simulink model "mainprevius"  (R2024b)
settings: Solver=VariableStepAuto  StartTime=0.0  StopTime=20  RelTol=1e-3
undefined symbols (not defined in the file or in its folder): ZigBee
libraries: truetime x11, fuzblock x2
settings Model: PacingRate=2  Creator=giovanni02  LastModifiedBy=Utente
settings ConfigComp: CovBoundaryAbsTol=1.0e-5

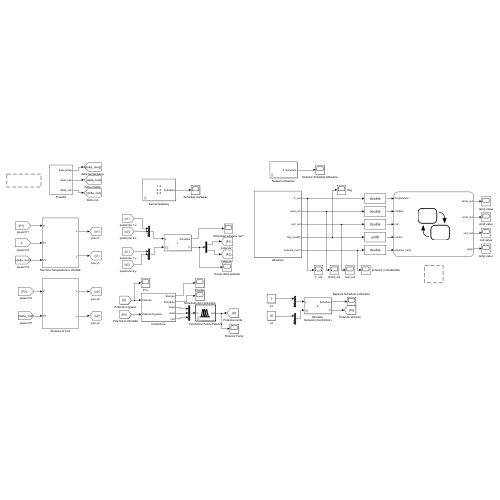
[thumbnail: Simulink's stored preview of the top-level diagram]
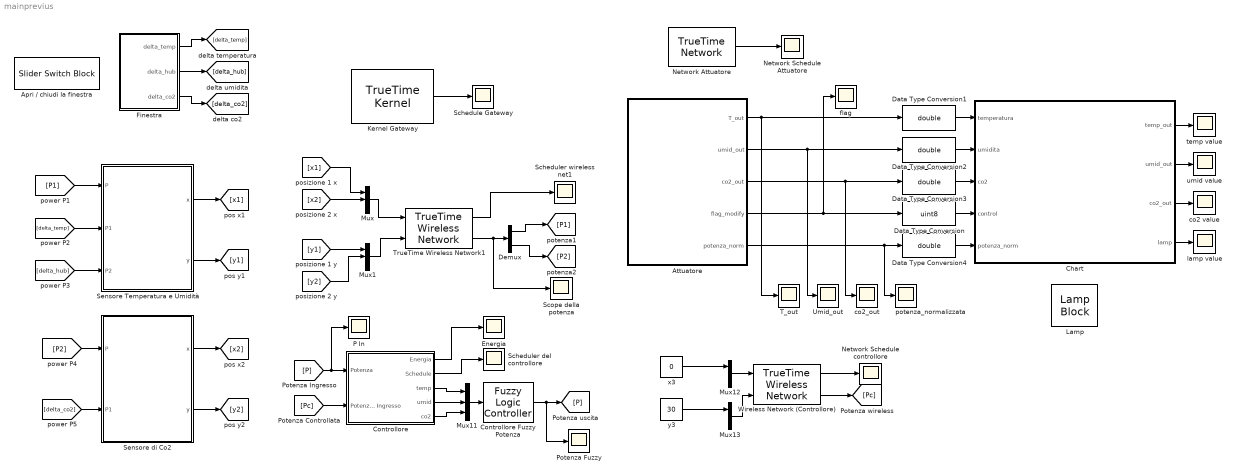
== system mainprevius ==
  Apri / chiudi la finestra : SliderSwitchBlock
      settings: Values={{'Off', 'On'}, [0 1]}
  Attuatore : Subsystem
  Chart : Stateflow chart  TreatAsAtomicUnit=on
      settings: PortSchema="{\"entries\":[{\"content\":{\"sides\":[{\"content\":{\"connectorIds\":[\"In2\",\"In3\",\"In4\",\"In1\",\"In5\"]},\"type\":\"ConnectorPlacement.EquallySpacedRectSide\",\"uuid\":\"3020dda5-3986-4acb-91a7-32414a76f8f2\"},{\"content\":{\"connectorIds\":[\"Out1\",\"Out2\",\"Out3\",\"Out4\"],\"side\":\"RIGHT\"},\"type\":\"ConnectorPlacement.EquallySpacedRectSide\",\"uuid\":\"ed764817-7f74-49da-be9c-3f2773007b92\"},{\"content\":{\"side\":\"TOP\"},\"type\":\"ConnectorPlacement.EquallySpacedRectSide\",\"uuid\":\"8abc556f-d358-4fb9-b14a-ffa987dc72f5\"}]},\"type\":\"ConnectorPlacement.EquallySpacedConnector\",\"uuid\":\"549e5bb5-9886-4c6a-8b6c-126bee32b5ab\"}],\"packageUris\":[\"http://schema.mathworks.com/mf0/Connector/R2020b\"],\"version\":\"1.0\"}"
  Controllore : Subsystem
  Controllore Fuzzy Potenza : fuzblock/Fuzzy Logic  Controller  FIS='ControlloreFuzzy.fis'  OutputSampleNumber=101  DataType=double  FuzzifiedInputs=off  RuleFiringStrengths=off  RuleOutputs=off  AggregatedOutputs=off  SimulateUsing=Interpreted execution  OutOfRangeInputValueMessage=warning  NoRuleFiredMessage=warning  EmptyOutputFuzzySetMessage=warning
  Data Type Conversion : DataTypeConversion  OutMin=[0]  OutMax=[5]  OutDataTypeStr=uint8  SaturateOnIntegerOverflow=off  RndMeth=Floor
  Data Type Conversion{1..4} (4 alike) : DataTypeConversion  OutMin=[0]  OutMax=[5]  OutDataTypeStr=double  SaturateOnIntegerOverflow=off  RndMeth=Floor
  Demux : Demux  Outputs=2
  Energia : Scope
  Finestra : Subsystem
  Kernel Gateway : truetime/TrueTime Kernel  sfun=Gateway_init  args=[]  ninputsoutputs=[0 0]  ntriggers=0  trigtype=falling  nwnodenbr=[1 4; 2 4; 3 4]  clockoffsetdrift=[0 0]  schedoutput=on  battery=off  poweroutput=off  label=1: 4\n2: 4\n3: 4
  Lamp : LampBlock  LabelPosition=Hide
  Mux : Mux  Inputs=3
  Mux1 : Mux  Inputs=3
  Mux11 : Mux  Inputs=3
  Mux12 : Mux  Inputs=2
  Mux13 : Mux  Inputs=2
  Network Attuatore : truetime/TrueTime Network  nwtype=CSMA/CD (Ethernet)  nwnbr=3  nnodes=4  rate=10000000  minsize=512  lossprob=0  seed=0  bandwidths=[0.5 0.5]  slotsize=512  schedule=[1 1 2]  memsize=80000  buftype=Common buffer  overflow=Retransmit  dynSchedule=0  miniSlotSize=0  NIT=0  QSortMode=FIFO  sync=0  irtSchedule=0  nrtLength=0  nodeGraph=0  scheduleoutput=on
  Network Schedule Attuatore : Scope
  Network Schedule controllore : Scope
  P In : Scope
  Potenza Fuzzy : Scope
  Schedule Gateway : Scope
  Scheduler del controllore : Scope
  Scheduler wireless net1 : Scope
  Scope della potenza : Scope
  Sensore Temperatura e Umidità : Subsystem
  Sensore di Co2 : Subsystem
  T_out : Scope
  TrueTime Wireless Network1 : truetime/TrueTime Wireless  Network  nwtype=802.15.4 (ZigBee)  nwnbr=1  nnodes=4  rate=800000  minsize=272  transpower=20  threshold=-48  use_pathloss_function=default  pathloss=3.5  acktimeout=0.00004  retrylimit=5  error_threshold=0.03  lossprob=0  seed=0  scheduleoutput=on  poweroutput=on
  Umid_out : Scope
  Wireless Network (Controllore) : truetime/TrueTime Wireless  Network  nwtype=802.15.4 (ZigBee)  nwnbr=2  nnodes=4  rate=800000  minsize=272  transpower=20  threshold=-48  use_pathloss_function=default  pathloss=3.5  acktimeout=0.00004  retrylimit=5  error_threshold=0.03  lossprob=0  seed=0  scheduleoutput=on  poweroutput=on
  co2 value : Scope
  co2_out : Scope
  flag : Scope
  lamp value : Scope
  potenza_normalizzata : Scope
  temp value : Scope
  umid value : Scope
  x3 : Constant  Value=0
  y3 : Constant  Value=30
  wires:
  [x2] -> Mux/2
  [y1] -> Mux1/1
  Mux/1 -> TrueTime Wireless Network1/1
  [y2] -> Mux1/2
  Mux1/1 -> TrueTime Wireless Network1/2
  Demux/1 -> [P1]
  TrueTime Wireless Network1/2 -> Scope della potenza/1, Demux/1
  [x1] -> Mux/1
  TrueTime Wireless Network1/1 -> Scheduler wireless net1/1
  Sensore Temperatura e Umidità/1(x) -> [x1]
  Sensore Temperatura e Umidità/2(y) -> [y1]
  [P1] -> Sensore Temperatura e Umidità/1(P)
  Finestra/2(delta_hub) -> [delta_hub]
  Finestra/1(delta_temp) -> [delta_temp]
  [delta_hub] -> Sensore Temperatura e Umidità/3(P2)
  [delta_temp] -> Sensore Temperatura e Umidità/2(P1)
  [P2] -> Sensore di Co2/1(P)
  [delta_co2] -> Sensore di Co2/2(P1)
  Sensore di Co2/1(x) -> [x2]
  Sensore di Co2/2(y) -> [y2]
  Finestra/3(delta_co2) -> [delta_co2]
  Demux/2 -> [P2]
  Kernel Gateway/1 -> Schedule Gateway/1
  [Pc] -> Controllore/2(Potenza Ingresso)
  Wireless Network (Controllore)/2 -> [Pc]
  x3/1 -> Mux12/1
  [P] -> P In/1, Controllore/1(Potenza)
  Wireless Network (Controllore)/1 -> Network Schedule controllore/1
  Mux13/1 -> Wireless Network (Controllore)/2
  Mux12/1 -> Wireless Network (Controllore)/1
  y3/1 -> Mux13/1
  Controllore Fuzzy Potenza/1 -> Potenza Fuzzy/1, [P]
  Mux11/1 -> Controllore Fuzzy Potenza/1
  Controllore/1(Energia) -> Energia/1
  Controllore/2(Schedule) -> Scheduler del controllore/1
  Controllore/3(temp) -> Mux11/1
  Attuatore/3(co2_out) -> Data Type Conversion3/1, co2_out/1
  Attuatore/2(umid_out) -> Umid_out/1, Data Type Conversion2/1
  Network Attuatore/1 -> Network Schedule Attuatore/1
  Attuatore/1(T_out) -> T_out/1, Data Type Conversion1/1
  Controllore/4(umid) -> Mux11/2
  Controllore/5(co2) -> Mux11/3
  Attuatore/4(flag_modify) -> flag/1, Data Type Conversion/1
  Data Type Conversion/1 -> Chart/1(control)
  Chart/4(lamp) -> lamp value/1
  Data Type Conversion3/1 -> Chart/4(co2)
  Data Type Conversion1/1 -> Chart/2(temperatura)
  Data Type Conversion2/1 -> Chart/3(umidita)
  Chart/1(temp_out) -> temp value/1
  Chart/2(umid_out) -> umid value/1
  Chart/3(co2_out) -> co2 value/1
  Attuatore/5(potenza_norm) -> potenza_normalizzata/1, Data Type Conversion4/1
  Data Type Conversion4/1 -> Chart/5(potenza_norm)

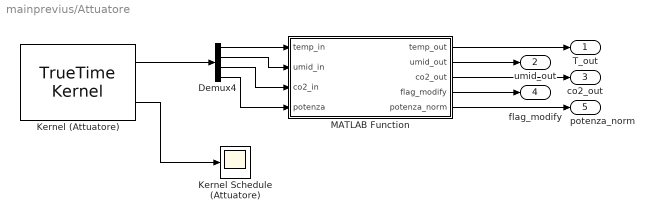
== system mainprevius/Attuatore ==
  Demux4 : Demux
  Kernel (Attuatore) : truetime/TrueTime Kernel  sfun=Attuatore_init  args=[]  ninputsoutputs=[0 4]  ntriggers=0  trigtype=falling  nwnodenbr=[3 1]  clockoffsetdrift=[0 0]  schedoutput=on  battery=off  poweroutput=off  label=3: 1
  Kernel Schedule (Attuatore) : Scope
  MATLAB Function : MATLAB Function  TreatAsAtomicUnit=on
  T_out : Outport
  umid_out : Outport  Port=2
  co2_out : Outport  Port=3
  flag_modify : Outport  Port=4
  potenza_norm : Outport  Port=5
  wires:
  Demux4/1 -> MATLAB Function/1(temp_in)
  Demux4/2 -> MATLAB Function/2(umid_in)
  Demux4/3 -> MATLAB Function/3(co2_in)
  Demux4/4 -> MATLAB Function/4(potenza)
  Kernel (Attuatore)/2 -> Kernel Schedule (Attuatore)/1
  Kernel (Attuatore)/1 -> Demux4/1
  MATLAB Function/1(temp_out) -> T_out/1
  MATLAB Function/2(umid_out) -> umid_out/1
  MATLAB Function/3(co2_out) -> co2_out/1
  MATLAB Function/4(flag_modify) -> flag_modify/1
  MATLAB Function/5(potenza_norm) -> potenza_norm/1

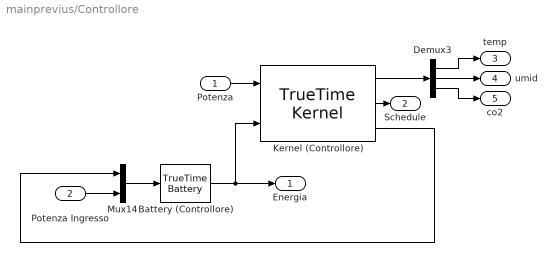
== system mainprevius/Controllore ==
  Potenza : Inport
  Potenza Ingresso : Inport  Port=2
  Battery (Controllore) : truetime/TrueTime Battery  energy=50
  Demux3 : Demux  Outputs=3
  Kernel (Controllore) : truetime/TrueTime Kernel  sfun=Controllore_init  args=[]  ninputsoutputs=[1 3]  ntriggers=0  trigtype=falling  nwnodenbr=[2 2]  clockoffsetdrift=[0 0]  schedoutput=on  battery=on  poweroutput=on  label=2: 2
  Mux14 : Mux  Inputs=2
  Energia : Outport
  Schedule : Outport  Port=2
  temp : Outport  Port=3
  umid : Outport  Port=4
  co2 : Outport  Port=5
  wires:
  Potenza Ingresso/1 -> Mux14/2
  Mux14/1 -> Battery (Controllore)/1
  Kernel (Controllore)/2 -> Schedule/1
  Potenza/1 -> Kernel (Controllore)/1
  Kernel (Controllore)/3 -> Mux14/1
  Kernel (Controllore)/1 -> Demux3/1
  Battery (Controllore)/1 -> Energia/1, Kernel (Controllore)/2
  Demux3/1 -> temp/1
  Demux3/3 -> co2/1
  Demux3/2 -> umid/1

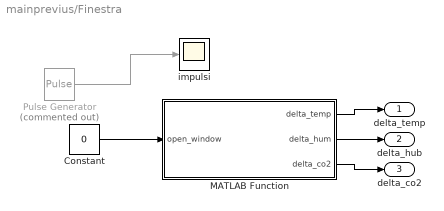
== system mainprevius/Finestra ==
  Constant : Constant  Value=0
  MATLAB Function : MATLAB Function  TreatAsAtomicUnit=on
  Pulse Generator : DiscretePulseGenerator  Commented=on  PulseType=Time based  Period=10  PulseWidth=5
  impulsi : Scope
  delta_temp : Outport
  delta_hub : Outport  Port=2
  delta_co2 : Outport  Port=3
  wires:
  Pulse Generator/1 -> impulsi/1
  MATLAB Function/1(delta_temp) -> delta_temp/1
  MATLAB Function/2(delta_hum) -> delta_hub/1
  MATLAB Function/3(delta_co2) -> delta_co2/1
  Constant/1 -> MATLAB Function/1(open_window)

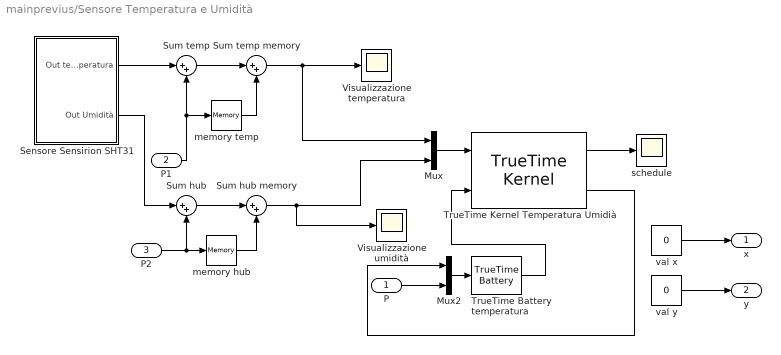
== system mainprevius/Sensore Temperatura e Umidità ==
  P : Inport
  P1 : Inport  Port=2
  P2 : Inport  Port=3
  Mux : Mux  Inputs=2
  Mux2 : Mux  Inputs=2
  "Sensore Sensirion SHT31 " : Subsystem
  Sum hub : Sum  Inputs=|++
  Sum hub memory : Sum  Inputs=|++
  Sum temp : Sum  Inputs=|++
  Sum temp memory : Sum  Inputs=|++
  TrueTime Battery temperatura : truetime/TrueTime Battery  energy=3
  TrueTime Kernel Temperatura Umidià : truetime/TrueTime Kernel  sfun=sensore_SensirionSHT31_init  args=[]  ninputsoutputs=[2 0]  ntriggers=0  trigtype=falling  nwnodenbr=[1 1]  clockoffsetdrift=[0 0]  schedoutput=on  battery=on  poweroutput=on  label=1: 1
  Visualizzazione temperatura : Scope
  Visualizzazione umidità : Scope
  memory hub : Memory
  memory temp : Memory
  schedule : Scope
  val x : Constant  Value=0
  val y : Constant  Value=0
  x : Outport
  y : Outport  Port=2
  wires:
  TrueTime Battery temperatura/1 -> TrueTime Kernel Temperatura Umidià/2
  val y/1 -> y/1
  P/1 -> Mux2/2
  TrueTime Kernel Temperatura Umidià/2 -> Mux2/1
  Sum temp memory/1 -> Mux/1, Visualizzazione temperatura/1
  Mux2/1 -> TrueTime Battery temperatura/1
  val x/1 -> x/1
  P1/1 -> Sum temp/2, memory temp/1
  memory hub/1 -> Sum hub memory/2
  "Sensore Sensirion SHT31 "/2(Out Umidità) -> Sum hub/1
  P2/1 -> Sum hub/2, memory hub/1
  memory temp/1 -> Sum temp memory/2
  "Sensore Sensirion SHT31 "/1(Out temperatura) -> Sum temp/1
  Sum temp/1 -> Sum temp memory/1
  Sum hub memory/1 -> Mux/2, Visualizzazione umidità/1
  Sum hub/1 -> Sum hub memory/1
  Mux/1 -> TrueTime Kernel Temperatura Umidià/1
  TrueTime Kernel Temperatura Umidià/1 -> schedule/1

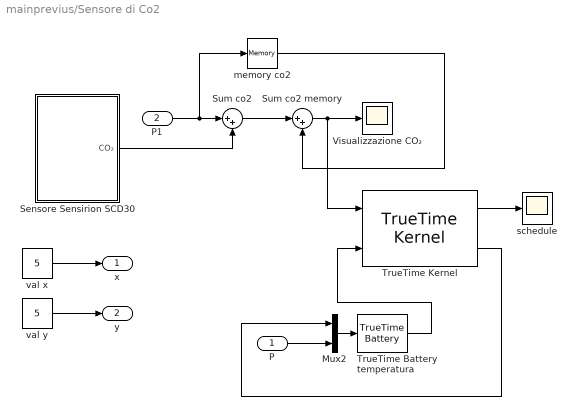
== system mainprevius/Sensore di Co2 ==
  P : Inport
  P1 : Inport  Port=2
  Mux2 : Mux  Inputs=2
  Sensore Sensirion SCD30 : Subsystem
  Sum co2 : Sum  Inputs=|++
  Sum co2 memory : Sum  Inputs=|++
  TrueTime Battery temperatura : truetime/TrueTime Battery  energy=3
  TrueTime Kernel : truetime/TrueTime Kernel  sfun=sensore_SensirionSCD30_init  args=[]  ninputsoutputs=[1 0]  ntriggers=0  trigtype=falling  nwnodenbr=[1 2]  clockoffsetdrift=[0 0]  schedoutput=on  battery=on  poweroutput=on  label=1: 2
  "Visualizzazione CO₂ " : Scope
  memory co2 : Memory
  schedule : Scope
  val x : Constant  Value=5
  val y : Constant  Value=5
  x : Outport
  y : Outport  Port=2
  wires:
  Sensore Sensirion SCD30/1("CO₂ ") -> Sum co2/2
  Sum co2/1 -> Sum co2 memory/1
  memory co2/1 -> Sum co2 memory/2
  P1/1 -> memory co2/1, Sum co2/1
  Sum co2 memory/1 -> TrueTime Kernel/1, "Visualizzazione CO₂ "/1
  TrueTime Battery temperatura/1 -> TrueTime Kernel/2
  val y/1 -> y/1
  val x/1 -> x/1
  P/1 -> Mux2/2
  TrueTime Kernel/2 -> Mux2/1
  TrueTime Kernel/1 -> schedule/1
  Mux2/1 -> TrueTime Battery temperatura/1

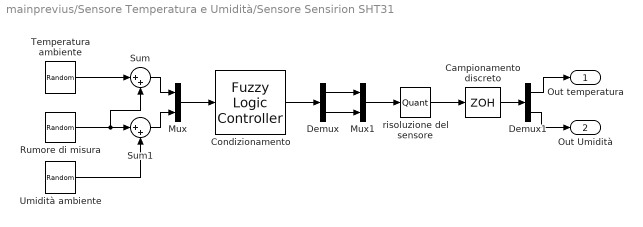
== system mainprevius/Sensore Temperatura e Umidità/Sensore Sensirion SHT31  ==
  Campionamento discreto : ZeroOrderHold  SampleTime=2
  Condizionamento : fuzblock/Fuzzy Logic  Controller  FIS='condizionamento.fis'  OutputSampleNumber=5  DataType=double  FuzzifiedInputs=off  RuleFiringStrengths=off  RuleOutputs=off  AggregatedOutputs=off  SimulateUsing=Interpreted execution  OutOfRangeInputValueMessage=warning  NoRuleFiredMessage=warning  EmptyOutputFuzzySetMessage=warning
  Demux : Demux  Outputs=2
  Demux1 : Demux  Outputs=2
  Mux : Mux  Inputs=2
  Mux1 : Mux  Inputs=2
  Rumore di misura : RandomNumber  Variance=2  Seed=2  SampleTime=200
  Sum : Sum  Inputs=|++
  Sum1 : Sum  Inputs=|++
  Temperatura ambiente : UniformRandomNumber  Minimum=15  Maximum=37  SampleTime=5
  Umidità ambiente : UniformRandomNumber  Minimum=0  Maximum=100  Seed=2  SampleTime=5
  risoluzione del sensore : Quantizer  QuantizationInterval=0.1
  Out temperatura : Outport
  Out Umidità : Outport  Port=2
  wires:
  Temperatura ambiente/1 -> Sum/1
  risoluzione del sensore/1 -> Campionamento discreto/1
  Demux1/2 -> Out Umidità/1
  Umidità ambiente/1 -> Sum1/2
  Rumore di misura/1 -> Sum/2, Sum1/1
  Mux/1 -> Condizionamento/1
  Sum1/1 -> Mux/2
  Sum/1 -> Mux/1
  Condizionamento/1 -> Demux/1
  Demux/1 -> Mux1/1
  Demux/2 -> Mux1/2
  Mux1/1 -> risoluzione del sensore/1
  Campionamento discreto/1 -> Demux1/1
  Demux1/1 -> Out temperatura/1

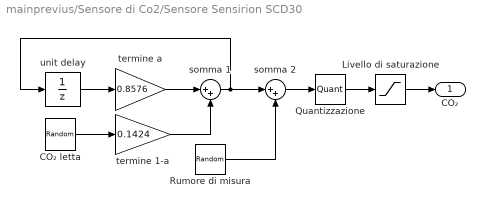
== system mainprevius/Sensore di Co2/Sensore Sensirion SCD30 ==
  CO₂ letta : UniformRandomNumber  Minimum=800  Maximum=1200  SampleTime=1
  Livello di saturazione : Saturate  UpperLimit=10000  LowerLimit=800
  Quantizzazione : Quantizer  QuantizationInterval=2
  Rumore di misura : RandomNumber  Variance=900  Seed=2  SampleTime=10
  somma 1 : Sum  Inputs=|++
  somma 2 : Sum  Inputs=|++
  termine 1-a : Gain  Gain=0.1424
  termine a : Gain  Gain=0.8576
  unit delay : UnitDelay  InitialCondition=1000  SampleTime=-1  HasFrameUpgradeWarning=on
  "CO₂ " : Outport
  wires:
  somma 1/1 -> somma 2/1, unit delay/1
  Quantizzazione/1 -> Livello di saturazione/1
  Livello di saturazione/1 -> "CO₂ "/1
  termine 1-a/1 -> somma 1/2
  CO₂ letta/1 -> termine 1-a/1
  unit delay/1 -> termine a/1
  termine a/1 -> somma 1/1
  somma 2/1 -> Quantizzazione/1
  Rumore di misura/1 -> somma 2/2

== matlab function mainprevius/Attuatore/MATLAB Function ==
  data: temp_in input; temp_out output; umid_in input; co2_in input; potenza input; umid_out output; co2_out output; flag_modify output; potenza_norm output
function [temp_out, umid_out, co2_out, flag_modify, potenza_norm] = fcn(temp_in, umid_in, co2_in, potenza)
temp_out = temp_in;
umid_out = umid_in;
co2_out = co2_in;

if potenza < 30
    flag_modify = 0;
elseif potenza >= 30 && potenza < 50
    flag_modify = 1;
else
    flag_modify = 2;
end

potenza_norm = potenza / 100;

== stateflow chart mainprevius/Chart ==
  state Stato1
    lamp = 0;
    temp_out = temperatura;
    umid_out = umidita;
    co2_out = co2;
  state Stato2
    lamp = 1;
    temp_out = temperatura;
    umid_out = umidita;
    co2_out = co2;
  state Stato0
    lamp = 0;
    temp_out = temperatura;
    umid_out = umidita;
    co2_out = co2;
  state Stato3
    lamp = 2;
    temp_out = temperatura;
    umid_out = umidita;
    co2_out = co2;
  Stato0 -> Stato1 [order 1] : [control < 0]
  Stato2 -> Stato1 [order 1] : [control < 0]
  Stato1 -> Stato2 : [control >= 0 && control <= 1]
  (default) -> Stato0
  Stato0 -> Stato2 [order 2] : [control >= 0 && control <= 1]
  Stato0 -> Stato3 [order 3] : [control > 1]
  Stato3 -> Stato2 : [control >= 0 && control <= 1]
  Stato2 -> Stato3 [order 2] : [control > 1]
  data: temp_out output double; control input uint8; umid_out output double; temperatura input double; umidita input double; co2 input double; co2_out output double; lamp output uint8; potenza_norm input double

== matlab function mainprevius/Finestra/MATLAB Function ==
  data: open_window input; delta_temp output; delta_hum output; delta_co2 output
function [delta_temp, delta_hum, delta_co2] = fcn(open_window)
% fcn: calcola la variazione (delta) di temperatura e umidità
% open_window = 1 -> finestra aperta
% open_window = 0 -> finestra chiusa

if open_window == 1
    % Finestra aperta: grande scambio termico con l'esterno
    delta_temp = - (1.5 + rand*1.0);   % abbassa temperatura di 1.5–2.5 °C
    delta_hum  =   (5 + rand*5);       % aumenta umidità di 5–10 %
    delta_co2 = - (50 + rand * 100);   % CO₂ cala rapidamente (aria fresca entra)
else
    % Finestra chiusa: accumulo termico e aria più secca
    delta_temp =  (0.3 + rand*0.2);    % aumenta temperatura di 0.3–0.5 °C
    delta_hum  = - (2 + rand*3);       % cala umidità di 2–5 %
    delta_co2 =   (5 + rand * 20);     % CO₂ cresce lentamente
end
end
